simulink model "sim_3D"  (R2020a)
settings: Solver=ode5  StartTime=0.0  StopTime=120  FixedStep=0.01  RelTol=1e-3  EnableMultiTasking=on
InitFcn:
  | python_config
  | load('simulation_parameters');
settings Model: ExtModeTrigMode=oneshot  ExtModeArmWhenConnect=off  Creator=laurensvaneykeren  LastModifiedBy=kdally
settings DataIOCC: SaveFormat=Array  SignalLoggingSaveFormat=ModelDataLogs  ReturnWorkspaceOutputs=off  SignalLoggingName=sigsOut
settings OptimizationCC: BooleanDataType=off  DefaultParameterBehavior=Inlined  EnhancedBackFolding=on  PassReuseOutputArgsAs=Individual arguments  ExpressionDepthLimit=2147483647  ZeroExternalMemoryAtStartup=off  ZeroInternalMemoryAtStartup=off  OptimizeBlockOrder=speed  DifferentSizesBufferReuse=on  OptimizationCustomize=off  EfficientTunableParamExpr=on
settings DebuggingCC: SaveWithParameterizedLinksMsg=none  UnderspecifiedInitializationDetection=Classic  MergeDetectMultiDrivingBlocksExec=none  SignalResolutionControl=TryResolveAllWithWarning  MultiTaskDSMMsg=warning  MultiTaskCondExecSysMsg=none  ParameterTunabilityLossMsg=error  FcnCallInpInsideContextMsg=warning  StateNameClashWarn=warning  SFUnexpectedBacktrackingDiag=warning  SFNoUnconditionalDefaultTransitionDiag=warning  SFExecutionAtInitializationDiag=none  ArithmeticOperatorsInVariantConditions=warning
settings HardwareCC: ProdBitPerPointer=32  ProdBitPerSizeT=32  ProdBitPerPtrDiffT=32  ProdLargestAtomicFloat=None  ProdIntDivRoundTo=Undefined  ProdEndianess=Unspecified  ProdWordSize=32  ProdHWDeviceType=32-bit Generic  TargetBitPerLong=64  TargetBitPerPointer=64  TargetBitPerSizeT=64  TargetBitPerPtrDiffT=64  TargetLongLongMode=on  TargetIntDivRoundTo=Zero  TargetEndianess=LittleEndian  TargetWordSize=64  TargetHWDeviceType=MATLAB Host  ProdEqTarget=off
settings ModelReferenceCC: PropagateSignalLabelsOutOfModel=off
settings SFSimCC: SimUseLocalCustomCode=off  MATLABDynamicMemAlloc=off  CustomCodeUndefinedFunction=UseInterfaceOnly
settings RTWCC: SystemTargetFile=ert.tlc  GenCodeOnly=on  TemplateMakefile=ert_default_tmf  GenerateReport=on  RTWUseLocalCustomCode=off  BuildConfiguration=Faster Runs
settings CodeAppCC: ForceParamTrailComments=on  IgnoreCustomStorageClasses=off  OperatorAnnotations=on  SimulinkDataObjDesc=on  SFDataObjDesc=on  InsertBlockDesc=on
settings ERTTargetCC: GenerateSampleERTMain=on  SupportContinuousTime=on  SupportNonInlinedSFcns=on  InlinedParameterPlacement=NonHierarchical  ERTCustomFileTemplate=example_file_process.tlc
settings ConfigComp: CovMetricSettings=dw  CovHtmlReporting=on  CovSaveCumulativeToWorkspaceVar=on  CovSaveSingleToWorkspaceVar=on  CovExternalEMLEnable=off

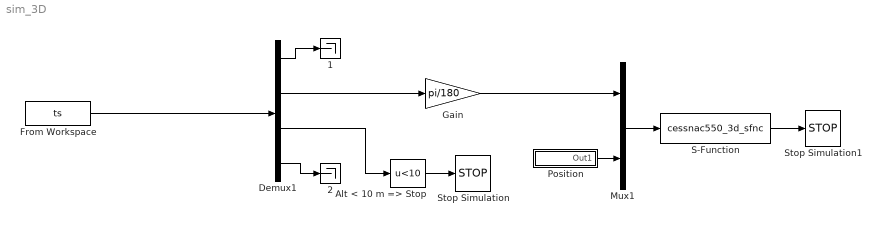
== system sim_3D ==
  1 : Terminator
  2 : Terminator
  Alt < 10 m => Stop : Fcn  Expr=u<10
  Demux1 : Demux  Outputs=[6 3 1 2]
      settings: DisplayOption=none
  From Workspace : FromWorkspace  VariableName=ts  SampleTime=-1  Interpolate=off  OutputAfterFinalValue=Holding final value
  Gain : Gain  Gain=pi/180
  Mux1 : Mux  Inputs=2
  Position : Subsystem
  S-Function : S-Function  FunctionName=cessnac550_3d_sfnc  SFunctionDeploymentMode=off  EnableBusSupport=off
  Stop Simulation : Stop
  Stop Simulation1 : Stop
  wires:
  Alt < 10 m => Stop/1 -> Stop Simulation/1
  Demux1/1 -> 1/1
  From Workspace/1 -> Demux1/1
  S-Function/1 -> Stop Simulation1/1
  Mux1/1 -> S-Function/1
  Demux1/4 -> 2/1
  Demux1/3 -> Alt < 10 m => Stop/1
  Position/1(Out1) -> Mux1/2
  Demux1/2 -> Gain/1
  Gain/1 -> Mux1/1

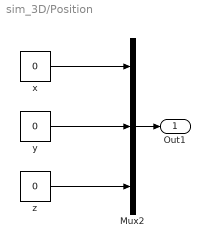
== system sim_3D/Position ==
  Mux2 : Mux  Inputs=3
  x : Constant  Value=0
  y : Constant  Value=0
  z : Constant  Value=0
  Out1 : Outport  VectorParamsAs1DForOutWhenUnconnected=off
  wires:
  y/1 -> Mux2/2
  z/1 -> Mux2/3
  x/1 -> Mux2/1
  Mux2/1 -> Out1/1
